simulink subsystem "rss_Temp"  (R2023a)
settings: Solver=VariableStepAuto  StartTime=0.0  StopTime=10.0  RelTol=1e-3
undefined symbols (not defined in the file): Gu16_tMotoTemp_CUR_ADMotoTempADC_X, Gu16_tPCBTemp_CUR_ADPCBTempADC_X, Gu16_tPwrTubTemp_CUR_ADPwrTubTempADC_X, Gu8_tMotoTemp_CUR, Gu8_tPCBTemp_CUR, Gu8_tPwrTubTemp_CUR
settings Model: Creator=xiaoqiang.yuan  LastModifiedBy=xiaoqiang.yuan

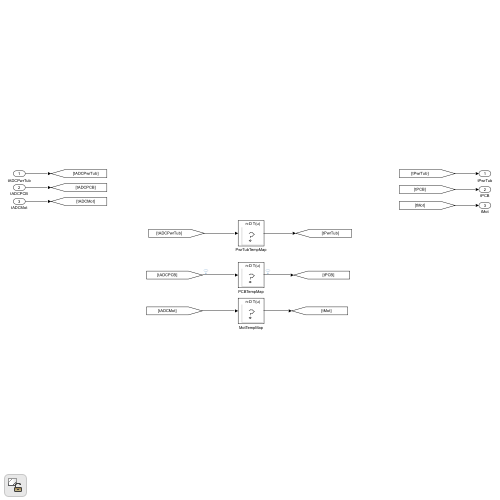
[thumbnail: Simulink's stored preview of the top-level diagram]
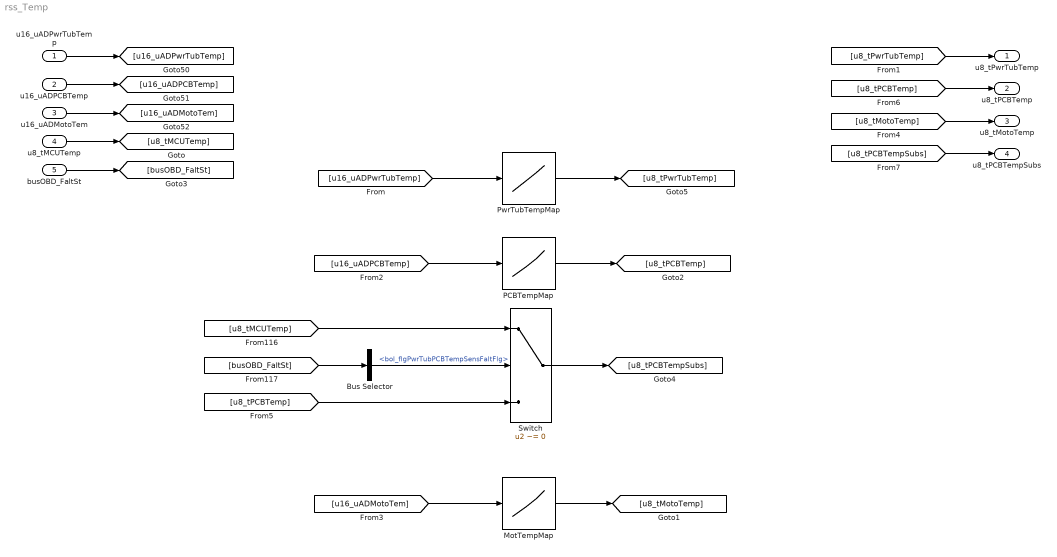
== system rss_Temp ==
  u16_uADPwrTubTemp : Inport  OutDataTypeStr=uint16
  u16_uADPCBTemp : Inport  Port=2  OutDataTypeStr=uint16
  u16_uADMotoTem : Inport  Port=3  OutDataTypeStr=uint16
  u8_tMCUTemp : Inport  Port=4  OutDataTypeStr=dt_Temp_u8p0bn40
  busOBD_FaltSt : Inport  Port=5  OutDataTypeStr=Bus: BUS_OBD_FALT_STS
  Bus Selector : BusSelector  OutputSignals=bol_flgPwrTubPCBTempSensFaltFlg
  MotTempMap : Lookup_n-D  NumberOfTableDimensions=1  BreakpointsForDimension1=Gu16_tMotoTemp_CUR_ADMotoTempADC_X  Table=Gu8_tMotoTemp_CUR  ExtrapMethod=Clip  InternalRulePriority=Speed  OutDataTypeStr=Inherit: Inherit from 'Table data'  RndMeth=Simplest
  PCBTempMap : Lookup_n-D  NumberOfTableDimensions=1  BreakpointsForDimension1=Gu16_tPCBTemp_CUR_ADPCBTempADC_X  Table=Gu8_tPCBTemp_CUR  ExtrapMethod=Clip  InternalRulePriority=Speed  OutDataTypeStr=Inherit: Inherit from 'Table data'  RndMeth=Simplest
  PwrTubTempMap : Lookup_n-D  NumberOfTableDimensions=1  BreakpointsForDimension1=Gu16_tPwrTubTemp_CUR_ADPwrTubTempADC_X  Table=Gu8_tPwrTubTemp_CUR  ExtrapMethod=Clip  InternalRulePriority=Speed  OutDataTypeStr=Inherit: Inherit from 'Table data'  RndMeth=Simplest
  Switch : Switch  Criteria=u2 ~= 0  SaturateOnIntegerOverflow=off  InputSameDT=off
  u8_tPwrTubTemp : Outport  OutDataTypeStr=dt_Temp_u8p0bn40
  u8_tPCBTemp : Outport  Port=2  OutDataTypeStr=dt_Temp_u8p0bn40
  u8_tMotoTemp : Outport  Port=3  OutDataTypeStr=dt_Temp_u8p0bn40
  u8_tPCBTempSubs : Outport  Port=4  OutDataTypeStr=dt_Temp_u8p0bn40
  wires:
  [u8_tPwrTubTemp] -> u8_tPwrTubTemp/1
  PwrTubTempMap/1 -> [u8_tPwrTubTemp]
  [u16_uADPwrTubTemp] -> PwrTubTempMap/1
  [u16_uADPCBTemp] -> PCBTempMap/1
  [u8_tPCBTemp] -> u8_tPCBTemp/1
  u16_uADPCBTemp/1 -> [u16_uADPCBTemp]
  u16_uADMotoTem/1 -> [u16_uADMotoTem]
  u16_uADPwrTubTemp/1 -> [u16_uADPwrTubTemp]
  MotTempMap/1 -> [u8_tMotoTemp]
  [u16_uADMotoTem] -> MotTempMap/1
  [u8_tMotoTemp] -> u8_tMotoTemp/1
  PCBTempMap/1 -> [u8_tPCBTemp]
  [busOBD_FaltSt] -> Bus Selector/1
  u8_tMCUTemp/1 -> [u8_tMCUTemp]
  busOBD_FaltSt/1 -> [busOBD_FaltSt]
  Bus Selector/1 -> Switch/2  "<bol_flgPwrTubPCBTempSensFaltFlg>"
  [u8_tMCUTemp] -> Switch/1
  [u8_tPCBTemp] -> Switch/3
  Switch/1 -> [u8_tPCBTempSubs]
  [u8_tPCBTempSubs] -> u8_tPCBTempSubs/1
